simulink model "esquematico_base"  (R2020a)
settings: Solver=VariableStepAuto  StartTime=0.0  StopTime=10.0  RelTol=1e-3
libraries: arduinolib x2
settings Model: Creator=Gloria Dani Abe  LastModifiedBy=Gloria Dani Abe

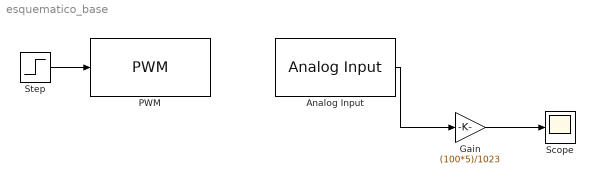
== system esquematico_base ==
  Analog Input : arduinolib/Analog Input  pinNumber=0  ReadResultsOnly=off  ConversionTriggerSource=Software  ExternalTriggerType=uint32( 0 )  OutputDataType=uint16  EnableConversionCompleteNotify=off  EnableOuputStatus=off  SampleTime=-1  blockPlatform=arduino
  Gain : Gain  Gain=(100*5)/1023
  PWM : arduinolib/PWM  pinNumber=13  frequencyType=Default  desiredFrequency=490.2  achievableFrequency=490.2
  Scope : Scope
  Step : Step  Before=(255*0)/100  After=(255*30)/100  SampleTime=0
  wires:
  Step/1 -> PWM/1
  Gain/1 -> Scope/1
  Analog Input/1 -> Gain/1
